simulink model "MCU_loggedData_dsPIC33CK_LVMC"  (R2023b)
settings: Solver=FixedStepDiscrete  StartTime=0.0  StopTime=10  FixedStep=50e-6  RelTol=1e-3
InitFcn:
  | % Sampling freq
  | Te = 0.5e-4 ;
  | 
  | % Electrical param
  | Rs = 0.6560; Ls = 3.5e-04;Ld = Ls; Lq = Ls; Phif= 0.0066;P= 4; Vemax=24;
  | 
  | % Mechanical param
  | J = 1e-5; f = 1e-5; Wrnom=2700*2*pi/60;
  | 
  | % State-space rep
  | A1c = [-Rs/(Ls) 0 ; 0 -Rs/(Ls)]; B1c= [1/(Ls) 0 ; 0 1/(Ls)]; C1c = [1 0 ; 0 1];
  | 
  | %Discretization
  | sys1d=c2d(ss(A1c, B1c, C1c, [0 0 ; 0 0]), Te, 'zoh');
  | [A1, B1, C1, D1]=ssdata(sys1d);
  | 
  | %DSMO param
  | h1 = 2/3; h2 = 15;
  | H1 = B1\A1*B1 + h1*eye(2); H2 = h2*eye(2); J_dsmo = [0 -1 ;  1 0];
  | 
  | % Adaptive obs param
  | gamma = 0.5/Te; h3 = 0.01; Telec = 2*pi/(Wrnom*P);fc = 3/(Telec);
undefined symbols (not defined in the file or in its folder): DiscIntNeverNeededParam, model
libraries: simulink x1
Description:
  | Offline real-time high frequency data logging based methodology
  | for PMSM observer design
  | 
  | Alhak Hassan et al.
  | ELECTRIMACS 2024 – Castello de la Plana, Spain, 27-30 May 2024
settings Model: Creator=rdelpoux  LastModifiedBy=rdelpoux

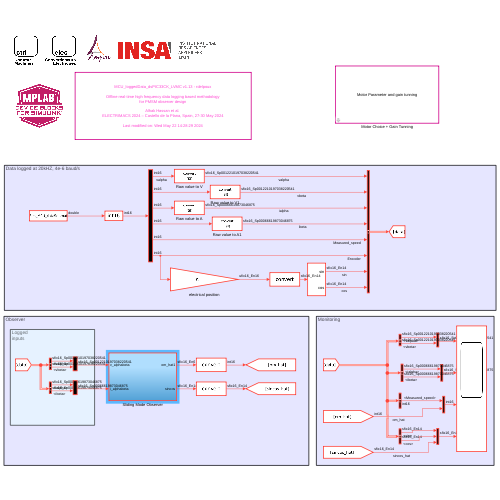
[thumbnail: Simulink's stored preview of the top-level diagram]
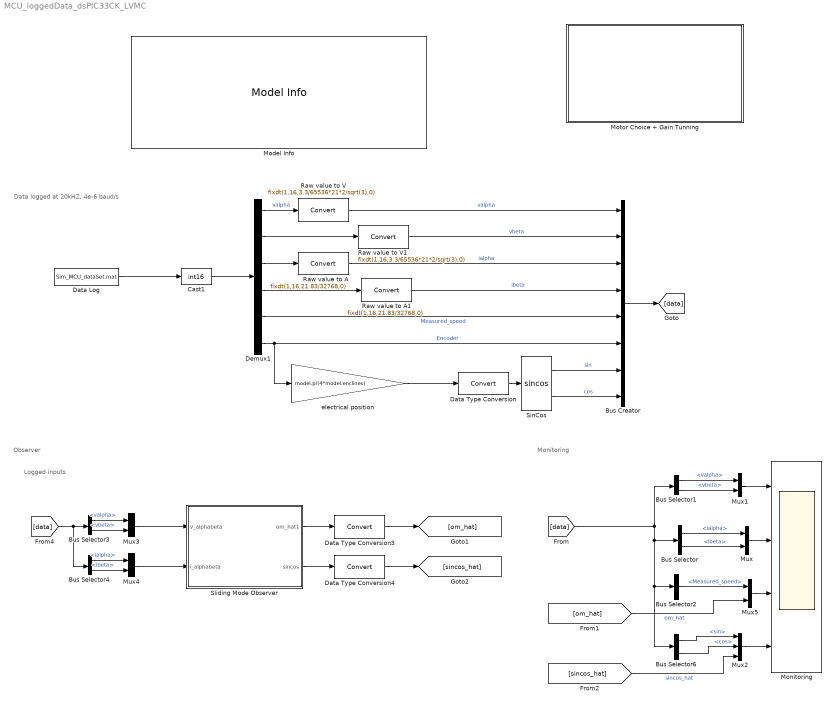
== system MCU_loggedData_dsPIC33CK_LVMC ==
  note: Logged
      | inputs
  note: Data logged at 20kHZ, 4e-6 baud/s
  note: Monitoring
  note: Observer
  Bus Creator : BusCreator  Inputs=8
  Bus Selector : BusSelector  OutputSignals=ialpha,ibeta
  Bus Selector1 : BusSelector  OutputSignals=valpha,vbeta
  Bus Selector2 : BusSelector  OutputSignals=Measured_speed
  Bus Selector3 : BusSelector  OutputSignals=valpha,vbeta
  Bus Selector4 : BusSelector  OutputSignals=ialpha,ibeta
  Bus Selector6 : BusSelector  OutputSignals=sin,cos
  Cast1 : DataTypeConversion  OutDataTypeStr=int16  SaturateOnIntegerOverflow=off  RndMeth=Floor
  Data Log : FromFile  FileName=Sim_MCU_dataSet.mat  SampleTime=50e-6
  Data Type Conversion : DataTypeConversion  SaturateOnIntegerOverflow=off  RndMeth=Floor
  Data Type Conversion3 : DataTypeConversion  SaturateOnIntegerOverflow=off  RndMeth=Floor
  Data Type Conversion4 : DataTypeConversion  SaturateOnIntegerOverflow=off  RndMeth=Floor
  Demux1 : Demux  Outputs=6
  Model Info : simulink/Model-Wide Utilities/Model Info  Frame=on  DisplayStringWithTags=|  HorizontalTextAlignment=Center  LeftAlignmentValue=0.5
      | %<ModelName> v%<ModelVersion> - %<Creator>
      | 
      | %<Description>
      | 
      | Last modified on: %<LastModificationDate>
  Monitoring : Scope  NumInputPorts=4
  Motor Choice + Gain Tunning : Subsystem  mask(INSA motor control gain tunning){presetMotor=Teknic-2310P, modelPMSM=Teknic-2310P, p=4, R=0.656, L=0.00035, Phif=0.0066, J=1e-05, F=1e-05, C0=0.01, vMax=48, iMax=10, omegaMax=500, enclines=1000, zetaE=0.7, trE=3*model.L/model.R, trWnE=3, KpE=0.2624, KiE=-1229.5314, zetaM=1.0, trM=0.05, trWnM=5, KpM=0.050253, KiM=-2.5253, tsMeca=1e-3}
      mask prompts: presetMotor "Predefined motor"; modelPMSM "PMSM model"; p "Poles pairs p"; R "Phase resistor R (Ohm)"; L "Phase inductance L (H)"; Phif "Flux constant Phif (Wb)"; J "Intertia J (kg.m^2)"; F "Damping coefficient F (N.m.s/rad)"; C0 "Coulomb friction C0 (N.m)"; vMax "Max Voltage (V)"; iMax "Max Current iMax (A)"; omegaMax "Max Speed (rad/s)"; enclines "Lines (RAW)"; zetaE "Damping factor (zeta)"; trE "Time response (s)"; trWnE "TrWn (3 for zeta = 0.7)"; KpE "Kp"; KiE "Ki"; zetaM "Damping factor (zeta)"; trM "Time response (s)"; trWnM "TrWn (3 for zeta = 0.7)"; KpM "Kp"; KiM "Ki"; tsMeca "Mecanical Sampling Time (s)"
      mask help: The bloc provides basic gain tunning solution based on pole placement.
      mask init:
      | % Mototor definition
      | model = struct;
      |          
      | switch presetMotor
      |     case 'Teknic-2310P'
      |         model.modelPMSM    = 'Teknic-2310P';                                 %           // Manufacturer Model Number
      |         model.p        = 4;                                                  %           // Pole Pairs for the motor
      |         model.R        = 0.656;                                              %Ohm        // Stator Resistor
      |         model.L        = 0.35e-3;                                            %H          // Inductance value
      |         model.Phif     = 6.6e-3;                                             %Wb         // PM flux
      |         model.J        = 1e-05;                                              %Kg-m2      // Inertia in SI units
      |         model.F        = 1.e-05;                                             %Kg-m2/s    // Friction Co-efficient
      |         model.C0       = 0.01;                                               %Kg-m2      // Dry friction
      |         model.vMax     = 48;                                                 %V          // Max voltage      
      |         model.iMax     = 10;                                                 %A          // Max current
      |         model.omegaMax = 500;                                                %rad/spm    // Max speed
      |         model.enclines = 1000;                                               % top       // Encoder top per round
      |     case 'Short HURST (AC300020)'
      |         model.modelPMSM    = 'Short HURST (AC300020)';                       %           // Manufacturer Model Number
      |         model.p        = 5;                                                  %           // Pole Pairs for the motor
      |         model.R        = 2.015;                                              %Ohm        // Stator Resistor
      |         model.L        = 2.3e-3;                                             %H          // Inductance value
      |         model.Phif     = 3.3e-3;                                             %Wb         // PM flux
      |         model.J        = 1.908e-04;                                          %Kg-m2      // Inertia in SI units
      |         model.F        = 1.044e-04;                                          %Kg-m2/s    // Friction Co-efficient
      |         model.C0       = 0.01;                                               %Kg-m2      // Dry friction
      |         model.vMax     = 48;                                                 %V          // Max voltage      
      |         model.iMax     = 10;                                                 %A          // Max current
      |         model.omegaMax = 350;                                                %rad/spm    // Max speed    
      |         model.enclines = NaN;                                                % top       // Encoder top per round
      |     case 'Long HURST (AC300022)'
      |         model.modelPMSM    = 'Long HURST (AC300022)';                        %           // Manufacturer Model Number
      |         model.p        = 5;                                                  %           // Pole Pairs for the motor
      |         model.R        = 0.405;                                              %Ohm        // Stator Resistor
      |         model.L        = 0.30e-3;                                            %H          // Inductance value
      |         model.Phif     = 7.63e-3;                                            %Wb         // PM flux
      |         model.J        = 1.908e-04;                                          %Kg-m2      // Inertia in SI units
      |         model.F        = 1.044e-04;                                          %Kg-m2/s    // Friction Co-efficient
      |         model.C0       = 0.01;                                               %Kg-m2      // Dry friction
      |         model.vMax     = 48;                                                 %V          // Max voltage      
      |         model.iMax     = 10;                                                 %A          // Max current
      |         model.omegaMax = 350;                                                %rad/spm    // Max speed    
      |         model.enclines = 250;                                                % top       // Encoder top per round
      |     case 'Custom'
      |         model.modelPMSM    = 'Custom';                                       %           // Manufacturer Model Number
      |         model.p        = p;                                                  %           // Pole Pairs for the motor
      |         model.R        = R;                                                  %Ohm        // Stator Resistor
      |         model.L        = L;                                                  %H          // Inductance value
      |         model.Phif     = Phif;                                               %Wb         // PM flux
      |         model.J        = J;                                                  %Kg-m2      // Inertia in SI units
      |         model.F        = F;                                                  %Kg-m2/s    // Friction Co-efficient
      |         model.C0       = C0;                                                 %Kg-m2      // Dry friction
      |         model.vMax     = vMax;                                               %V          // Max voltage      
      |         model.iMax     = iMax;                                               %A          // Max current
      |         model.omegaMax = omegaMax;                                           %rad/spm    // Max speed
      |         model.enclines = enclines;                                           % top       // Encoder top per round
      | end
      | 
      | 
      | 
      | ff = fields(model);
      | for i=1:numel(ff)
      |     set_param(gcb,ff{i},num2str(model.(ff{i})) );
      | end
      | %% Define fracation length for fixed point datatype
      | model.FracLen.curr  = (15-ceil(log2(model.iMax)));  % Fraction length for current variables
      | model.FracLen.volt  = (15-ceil(log2(model.vMax)));    % Fraction length for voltage variables
      | model.FracLen.volt2 = (15-ceil(log2(2*model.vMax^2))); % Fraction length for voltage square variables
      | model.FracLen.invsqrtvolt = (15-ceil(log2(1/sqrt(model.vMax/4)^2))); % Fraction length for voltage square variables
      | 
      | 
      | %% LUT 1/sqrt(||v_dq||)
      | func = '1./sqrt(x)';
      | xmin = (model.vMax/4)^2; xmax = 2*model.vMax^2;
      | 
      | xdt = sfix(16); xscale = 2^-(15-ceil(log2(xmax)));
      | ydt = sfix(16); yscale = 2^-(15-ceil(log2(1./sqrt(xmin))));
      | rndmeth = 'Floor';
      | errmax = [];
      | nptsmax = [128];
      | spacing = 'even';
      | 
      | %Compute LUT
      | [model.math.LUTintsqrtx,model.math.LUTintsqrty] = fixpt_look1_func_approx(func,xmin,xmax,xdt,xscale,ydt,yscale,rndmeth,errmax,nptsmax,spacing);
      | 
      | 
      | assignin('base','model',model);
      | 
      | %% Define control structure 
      | control = struct;
      | control.tauElec = model.L/model.R;
      | control.kElec = 1/model.R;
      | control.tauMeca = model.J/model.F;
      | control.kMeca = 3/2*model.p*model.Phif/model.F;
      | 
      | 
      | control.trDElec = trE;
      | control.zetaDElec = zetaE;
      | control.trwnDElec = trWnE;
      | control.wnDElec = control.trwnDElec/control.trDElec;
      | control.kE = [(2*control.zetaDElec*control.wnDElec*control.tauElec-1)/control.kElec, ...
      |                 -control.tauElec*control.wnDElec^2/control.kElec];
      | set_param(gcb, 'KpE', num2str(control.kE(1)));
      | set_param(gcb, 'KiE', num2str(control.kE(2)));
      | 
      | control.trDMeca = trM;
      | control.zetaDMeca = zetaM;
      | control.trwnDMeca = trWnM;
      | control.wnDMeca = control.trwnDMeca/control.trDMeca;
      | control.kM = [(2*control.zetaDMeca*control.wnDMeca*control.tauMeca-1)/control.kMeca, ...
      |                 -control.tauMeca*control.wnDMeca^2/control.kMeca];
      | set_param(gcb, 'KpM', num2str(control.kM(1)));
      | set_param(gcb, 'KiM', num2str(control.kM(2)));
      | 
      | control.tsMeca = tsMeca;
      | 
      | assignin('base','control',control);
      mask Help: For more help on the gain tunning, visit http://rcp.ctrl-elec.fr
      mask TypeOptions presetMotor: Custom | Teknic-2310P | Short HURST (AC300020) | Long HURST (AC300022)
      mask DialogControl DescGroupVar Prompt: Moteur Synchrone à aimants permanents
      mask DialogControl DescTextVar Prompt: Motor Parameters for gain tunning
      mask DialogControl Container4 Prompt: Motor Parameters
      mask DialogControl Container7 Prompt: Parameters
      mask DialogControl Container8 Prompt: Electrical parameters
      mask DialogControl Container9 Prompt: Mechanical parameters
      mask DialogControl Container13 Prompt: Motor Limits
      mask DialogControl Container14 Prompt: Encoder
      mask DialogControl Container10 Prompt: Gain Tuning
      mask DialogControl Control2 Prompt: Pole placement
      mask DialogControl Container11 Prompt: Electrical Dynamic
      mask DialogControl Container12 Prompt: Mechanical Dynamic
      mask Display: disp('Motor Parameter and gain tunning');
  Mux{,1,3..5} (5 alike) : Mux  Inputs=2
  Mux2 : Mux  Inputs=3
  Raw value to A : DataTypeConversion  OutDataTypeStr=fixdt(1,16,21.83/32768,0)  ConvertRealWorld=Stored Integer (SI)  SaturateOnIntegerOverflow=off  RndMeth=Floor
  Raw value to A1 : DataTypeConversion  OutDataTypeStr=fixdt(1,16,21.83/32768,0)  ConvertRealWorld=Stored Integer (SI)  SaturateOnIntegerOverflow=off  RndMeth=Floor
  Raw value to V : DataTypeConversion  OutDataTypeStr=fixdt(1,16,3.3/65536*21*2/sqrt(3),0)  ConvertRealWorld=Stored Integer (SI)  SaturateOnIntegerOverflow=off  RndMeth=Floor
  Raw value to V1 : DataTypeConversion  OutDataTypeStr=fixdt(1,16,3.3/65536*21*2/sqrt(3),0)  ConvertRealWorld=Stored Integer (SI)  SaturateOnIntegerOverflow=off  RndMeth=Floor
  SinCos : Trigonometry  Operator=sincos  ApproximationMethod=Lookup  AngleUnit=revolution  TableDataTypeStr=fixdt(1,16,14)
  Sliding Mode Observer : Subsystem
  electrical position : Gain  Gain=model.p/(4*model.enclines)  OutDataTypeStr=fixdt(0,16,16)
  wires:
  Bus Creator/1 -> [data]
  Bus Selector/1 -> Mux/1  "<ialpha>"
  Bus Selector/2 -> Mux/2  "<ibeta>"
  Mux1/1 -> Monitoring/1
  Bus Selector1/2 -> Mux1/2  "<vbeta>"
  Bus Selector1/1 -> Mux1/1  "<valpha>"
  [data] -> Bus Selector/1, Bus Selector6/1, Bus Selector2/1, Bus Selector1/1
  Demux1/5 -> Bus Creator/5  "Measured_speed"
  Data Log/1 -> Cast1/1
  Demux1/3 -> Raw value to A/1
  Demux1/4 -> Raw value to A1/1
  Demux1/2 -> Raw value to V1/1
  Demux1/1 -> Raw value to V/1  "valpha"
  Demux1/6 -> electrical position/1, Bus Creator/6  "Encoder"
  Mux/1 -> Monitoring/2
  Bus Selector2/1 -> Mux5/1  "<Measured_speed>"
  Bus Selector3/1 -> Mux3/1  "<valpha>"
  Bus Selector3/2 -> Mux3/2  "<vbeta>"
  Mux3/1 -> Sliding Mode Observer/1(v_alphabeta)
  [data] -> Bus Selector4/1, Bus Selector3/1
  Bus Selector4/2 -> Mux4/2  "<ibeta>"
  Bus Selector4/1 -> Mux4/1  "<ialpha>"
  Cast1/1 -> Demux1/1
  Raw value to V/1 -> Bus Creator/1  "valpha"
  Raw value to V1/1 -> Bus Creator/2  "vbeta"
  Raw value to A/1 -> Bus Creator/3  "ialpha"
  Raw value to A1/1 -> Bus Creator/4  "ibeta"
  electrical position/1 -> Data Type Conversion/1
  Data Type Conversion/1 -> SinCos/1
  SinCos/1 -> Bus Creator/7  "sin"
  SinCos/2 -> Bus Creator/8  "cos"
  Bus Selector6/1 -> Mux2/1  "<sin>"
  Bus Selector6/2 -> Mux2/2  "<cos>"
  Mux2/1 -> Monitoring/4
  Mux5/1 -> Monitoring/3
  [om_hat] -> Mux5/2  "om_hat"
  Mux4/1 -> Sliding Mode Observer/2(i_alphabeta)
  [sincos_hat] -> Mux2/3  "sincos_hat"
  Sliding Mode Observer/1(om_hat1) -> Data Type Conversion3/1
  Sliding Mode Observer/2(sincos) -> Data Type Conversion4/1
  Data Type Conversion3/1 -> [om_hat]
  Data Type Conversion4/1 -> [sincos_hat]

== system MCU_loggedData_dsPIC33CK_LVMC/Motor Choice + Gain Tunning ==

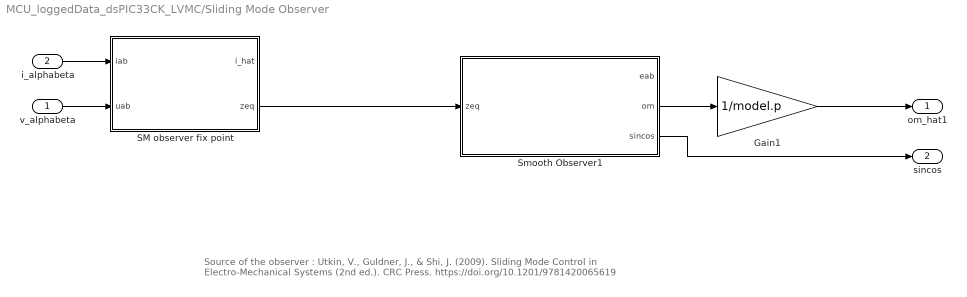
== system MCU_loggedData_dsPIC33CK_LVMC/Sliding Mode Observer ==
  note: Source of the observer : Utkin, V., Guldner, J., & Shi, J. (2009). Sliding Mode Control in Electro-Mechanical Systems (2nd ed.). CRC Press. https://doi.org/10.1201/9781420065619
  v_alphabeta : Inport
  i_alphabeta : Inport  Port=2
  Gain1 : Gain  Gain=1/model.p  OutMax=model.omegaMax  OutDataTypeStr=fixdt(1,16)
  SM observer fix point : Subsystem
  Smooth Observer1 : Subsystem
  om_hat1 : Outport
  sincos : Outport  Port=2
  wires:
  Smooth Observer1/3(sincos) -> sincos/1
  Gain1/1 -> om_hat1/1
  Smooth Observer1/2(om) -> Gain1/1
  v_alphabeta/1 -> SM observer fix point/2(uab)
  i_alphabeta/1 -> SM observer fix point/1(iab)
  SM observer fix point/2(zeq) -> Smooth Observer1/1(zeq)

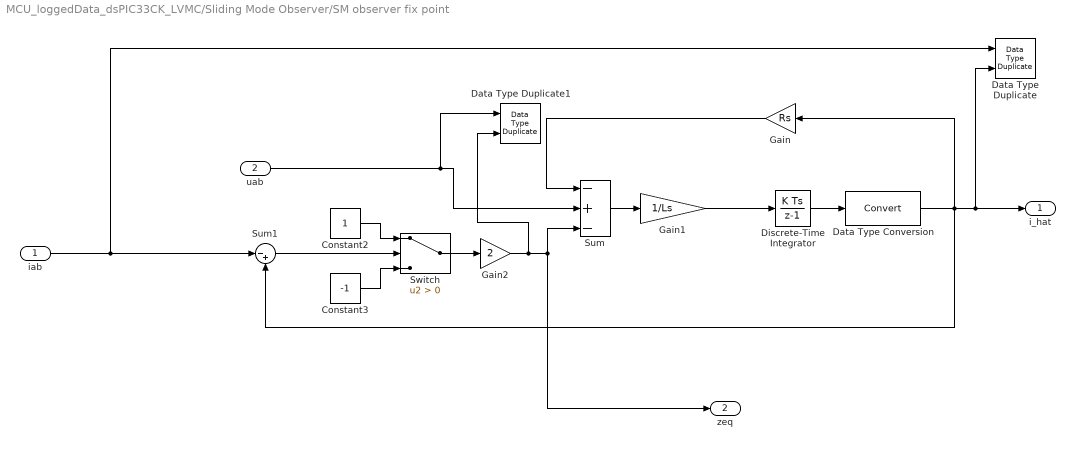
== system MCU_loggedData_dsPIC33CK_LVMC/Sliding Mode Observer/SM observer fix point ==
  iab : Inport
  uab : Inport  Port=2
  Constant2 : Constant  OutDataTypeStr=int16
  Constant3 : Constant  Value=-1  OutDataTypeStr=int16
  Data Type Duplicate : DataTypeDuplicate
  Data Type Duplicate1 : DataTypeDuplicate
  Data Type Conversion : DataTypeConversion  SaturateOnIntegerOverflow=off  RndMeth=Floor
  Discrete-Time Integrator : DiscreteIntegrator  SampleTime=-1  OutDataTypeStr=fixdt(1,32,10)  ICPrevOutput=DiscIntNeverNeededParam  ICPrevScaledInput=DiscIntNeverNeededParam
  Gain : Gain  Gain=Rs  OutDataTypeStr=Inherit: Same as input
  Gain1 : Gain  Gain=1/Ls  OutDataTypeStr=Inherit: Same as input
  Gain2 : Gain  Gain=2  OutMax=[10]  OutDataTypeStr=Inherit: Inherit via back propagation
  Sum : Sum  Inputs=-+-  OutDataTypeStr=fixdt(1,32,10)
  Sum1 : Sum  Inputs=|-+
  Switch : Switch  Criteria=u2 > Threshold  SaturateOnIntegerOverflow=off  InputSameDT=off
  i_hat : Outport  VectorParamsAs1DForOutWhenUnconnected=off
  zeq : Outport  Port=2  VectorParamsAs1DForOutWhenUnconnected=off
  wires:
  Data Type Conversion/1 -> Gain/1, i_hat/1, Data Type Duplicate/2, Sum1/2
  Sum/1 -> Gain1/1
  Gain/1 -> Sum/1
  uab/1 -> Data Type Duplicate1/1, Sum/2
  Gain2/1 -> Data Type Duplicate1/2, zeq/1, Sum/3
  Switch/1 -> Gain2/1
  Discrete-Time Integrator/1 -> Data Type Conversion/1
  Gain1/1 -> Discrete-Time Integrator/1
  iab/1 -> Sum1/1, Data Type Duplicate/1
  Constant3/1 -> Switch/3
  Sum1/1 -> Switch/2
  Constant2/1 -> Switch/1

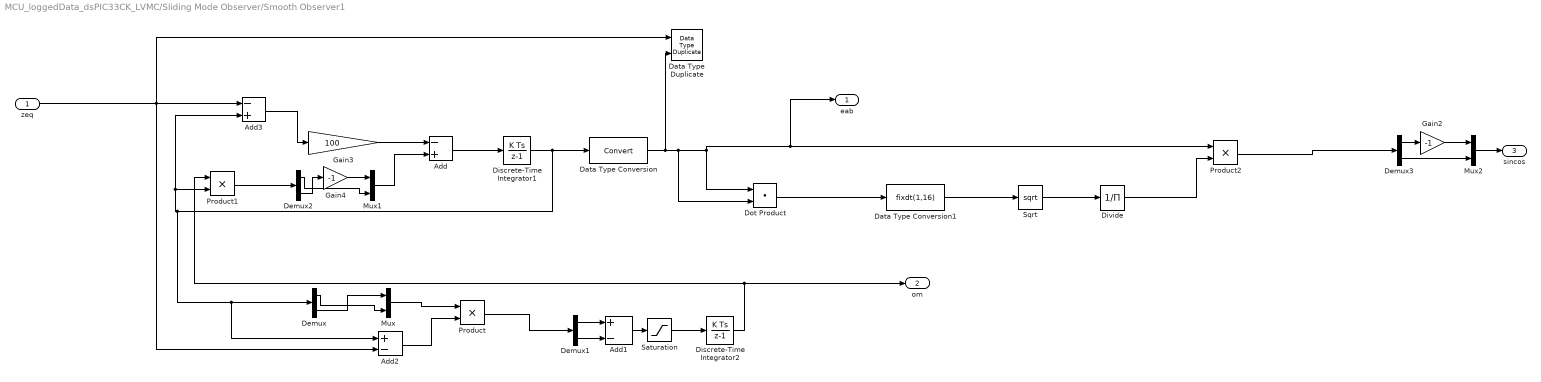
== system MCU_loggedData_dsPIC33CK_LVMC/Sliding Mode Observer/Smooth Observer1 ==
  zeq : Inport
  Add : Sum  Inputs=-+  OutDataTypeStr=Inherit: Same as first input
  Add1 : Sum  Inputs=+-  OutDataTypeStr=Inherit: Same as first input
  Add2 : Sum  Inputs=+-
  Add3 : Sum  Inputs=-+  OutDataTypeStr=fixdt(1,32,10)
  Data Type Duplicate : DataTypeDuplicate
  Data Type Conversion : DataTypeConversion  SaturateOnIntegerOverflow=off  RndMeth=Floor
  Data Type Conversion1 : DataTypeConversion  OutMax=[model.vMax^2]  OutDataTypeStr=fixdt(1,16)  SaturateOnIntegerOverflow=off  RndMeth=Floor
  Demux{,1..3} (4 alike) : Demux  Outputs=2
  Discrete-Time Integrator1 : DiscreteIntegrator  SampleTime=-1  OutDataTypeStr=fixdt(1,32,10)  ICPrevOutput=DiscIntNeverNeededParam  ICPrevScaledInput=DiscIntNeverNeededParam
  Discrete-Time Integrator2 : DiscreteIntegrator  gainval=8000  SampleTime=-1  OutDataTypeStr=fixdt(1,32,10)  ICPrevOutput=DiscIntNeverNeededParam  ICPrevScaledInput=DiscIntNeverNeededParam
  Divide : Product  Inputs=/  OutMax=[1]  OutDataTypeStr=fixdt(1,16)  SaturateOnIntegerOverflow=on
  Dot Product : DotProduct  SaturateOnIntegerOverflow=on
  Gain2 : Gain  Gain=-1  OutDataTypeStr=Inherit: Same as input  ParamDataTypeStr=Inherit: Same as input
  Gain3 : Gain  Gain=100  OutDataTypeStr=Inherit: Same as input
  Gain4 : Gain  Gain=-1  OutDataTypeStr=Inherit: Same as input
  Mux : Mux  Inputs=2
  Mux1 : Mux  Inputs=2
  Mux2 : Mux  Inputs=2
  Product : Product  OutDataTypeStr=Inherit: Same as first input
  Product1 : Product  OutDataTypeStr=Inherit: Same as first input
  Product2 : Product  OutMax=[1]  OutDataTypeStr=fixdt(1,16)
  Saturation : Saturate  UpperLimit=1  LowerLimit=-1
  Sqrt : Sqrt
  eab : Outport  VectorParamsAs1DForOutWhenUnconnected=off
  om : Outport  Port=2  VectorParamsAs1DForOutWhenUnconnected=off
  sincos : Outport  Port=3  VectorParamsAs1DForOutWhenUnconnected=off
  wires:
  Gain2/1 -> Mux2/1
  Demux3/2 -> Mux2/2
  Demux3/1 -> Gain2/1
  Mux2/1 -> sincos/1
  Divide/1 -> Product2/2
  Product2/1 -> Demux3/1
  Sqrt/1 -> Divide/1
  Dot Product/1 -> Data Type Conversion1/1
  Demux2/2 -> Gain4/1
  Product/1 -> Demux1/1
  Demux/2 -> Mux/1
  Demux1/2 -> Add1/2
  Add/1 -> Discrete-Time Integrator1/1
  Gain4/1 -> Mux1/1
  Demux1/1 -> Add1/1
  Demux/1 -> Mux/2
  Demux2/1 -> Mux1/2
  Product1/1 -> Demux2/1
  Gain3/1 -> Add/1
  Mux/1 -> Product/1
  Add1/1 -> Saturation/1
  Mux1/1 -> Add/2
  Add3/1 -> Gain3/1
  Add2/1 -> Product/2
  Discrete-Time Integrator1/1 -> Data Type Conversion/1, Add3/2, Product1/2, Add2/1, Demux/1
  Saturation/1 -> Discrete-Time Integrator2/1
  Discrete-Time Integrator2/1 -> Product1/1, om/1
  Data Type Conversion/1 -> Data Type Duplicate/2, Dot Product/1, Product2/1, eab/1, Dot Product/2
  Data Type Conversion1/1 -> Sqrt/1
  zeq/1 -> Data Type Duplicate/1, Add3/1, Add2/2
